simulink model "Sim_exe"  (R2020b)
settings: Solver=VariableStepAuto  StartTime=0.0  StopTime=Tf  RelTol=1e-4  AbsTol=1e-4
values from neighbouring files (symbols this model uses):
  C = [0,1]    [Main.m]
  IC_kf = zeros(2,1)    [Main.m]
  Namp = 1*10^-1    (= 0.1)    [Main.m]
  Qk = 1    [Main.m]
  Rk = 1    [Main.m]
  Tf = T(end)    [Main.m]
  Wamp = 0*5e-3    (= 0)    [Main.m]
settings Model: Creator=emanuele riva  LastModifiedBy=emanu
settings SolverCC: AutoScaleAbsTol=off
settings DataIOCC: ReturnWorkspaceOutputs=off
settings DebuggingCC: ArithmeticOperatorsInVariantConditions=warning
settings SFSimCC: SimUseLocalCustomCode=off  CustomCodeUndefinedFunction=UseInterfaceOnly
settings RTWCC: RTWUseLocalCustomCode=off
settings CodeAppCC: StateflowObjectComments=on

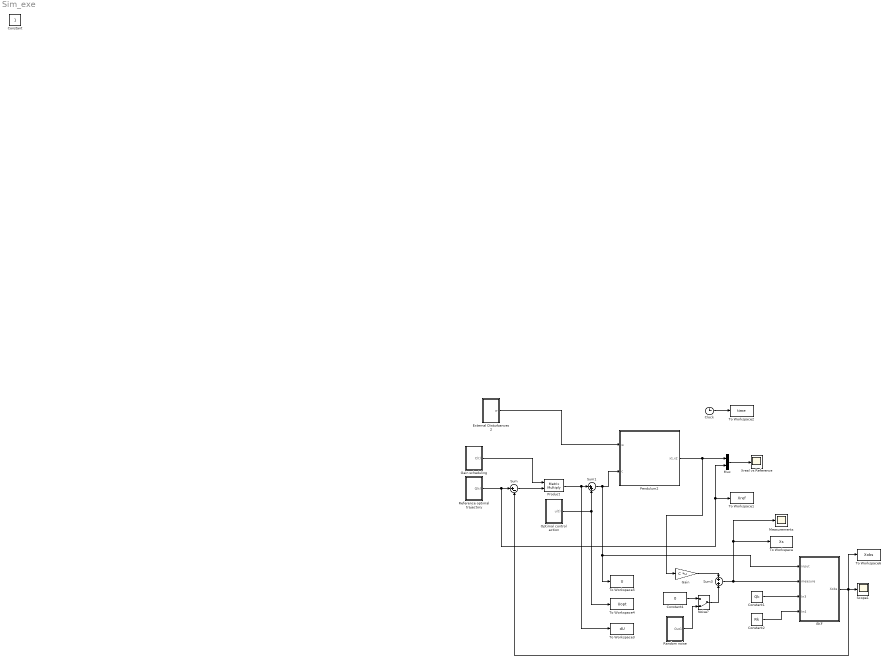
== system Sim_exe ==
  Clock : Clock
  Constant1 : Constant  Value=Qk
  Constant2 : Constant  Value=Rk
  Constant4 : Constant  Value=0
  EKF : Subsystem
  External Disturbances2 : Subsystem
  Gain : Gain  Gain=C  Multiplication=Matrix(K*u)
  Gain scheduling : Subsystem
  Measurements : Scope
  Mux : Mux  Inputs=2
  Noise? : ManualSwitch  CurrentSetting=0
  Optimal control action : Subsystem
  Pendulum2 : Subsystem
  Product : Product  Multiplication=Matrix(*)
  Random noise : Subsystem
  Reference optimal trajectory : Subsystem
  Scope1 : Scope
  Sum : Sum  Inputs=|+-
  Sum1 : Sum  Inputs=|++
  Sum3 : Sum
  To Workspace : ToWorkspace  VariableName=Xs  SaveFormat=Timeseries  SampleTime=-1
  To Workspace1 : ToWorkspace  VariableName=Xref  SaveFormat=Timeseries  SampleTime=-1
  To Workspace2 : ToWorkspace  VariableName=time  SaveFormat=Timeseries  SampleTime=-1
  To Workspace3 : ToWorkspace  VariableName=dU  SaveFormat=Timeseries  SampleTime=-1
  To Workspace4 : ToWorkspace  VariableName=Uopt  SaveFormat=Timeseries  SampleTime=-1
  To Workspace5 : ToWorkspace  VariableName=U  SaveFormat=Timeseries  SampleTime=-1
  To Workspace6 : ToWorkspace  VariableName=Xobs  SaveFormat=Timeseries  SampleTime=-1
  Xreal vs Reference : Scope
  Constant : Constant  IOType=siggen
  wires:
  Pendulum2/1(x1,x2) -> Gain/1, Mux/1
  Reference optimal trajectory/1(Q(t)) -> Mux/2, To Workspace1/1, Sum/1
  Gain scheduling/1(C(t)) -> Product/1
  Sum/1 -> Product/2
  Product/1 -> Sum1/1, To Workspace3/1
  Optimal control action/1(u(t)) -> To Workspace4/1, Sum1/2
  Mux/1 -> Xreal vs Reference/1
  Clock/1 -> To Workspace2/1
  Constant1/1 -> EKF/3(In3)
  Constant2/1 -> EKF/4(In4)
  EKF/1(Xobs) -> To Workspace6/1, Sum/2, Scope1/1
  Constant4/1 -> Noise?/1
  Random noise/1(Out1) -> Noise?/2
  Noise?/1 -> Sum3/2
  Gain/1 -> Sum3/1
  Sum3/1 -> To Workspace/1, Measurements/1, EKF/2(measure)
  Sum1/1 -> Pendulum2/2(c), To Workspace5/1, EKF/1(input)
  External Disturbances2/1(w) -> Pendulum2/1(w)

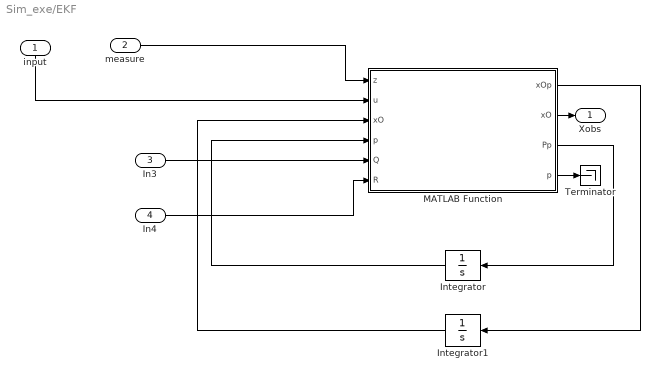
== system Sim_exe/EKF ==
  input : Inport
  measure : Inport  Port=2
  In3 : Inport  Port=3
  In4 : Inport  Port=4
  Integrator : Integrator  InitialCondition=zeros(4,1)
  Integrator1 : Integrator  InitialCondition=IC_kf
  MATLAB Function : MATLAB Function  TreatAsAtomicUnit=on
  Terminator : Terminator
  Xobs : Outport
  wires:
  MATLAB Function/1(xOp) -> Integrator1/1
  Integrator1/1 -> MATLAB Function/3("xO ")
  MATLAB Function/2(xO) -> Xobs/1
  MATLAB Function/4(p) -> Terminator/1
  input/1 -> MATLAB Function/2(u)
  In4/1 -> MATLAB Function/6(R)
  Integrator/1 -> MATLAB Function/4("p ")
  In3/1 -> MATLAB Function/5(Q)
  measure/1 -> MATLAB Function/1(z)
  MATLAB Function/3(Pp) -> Integrator/1

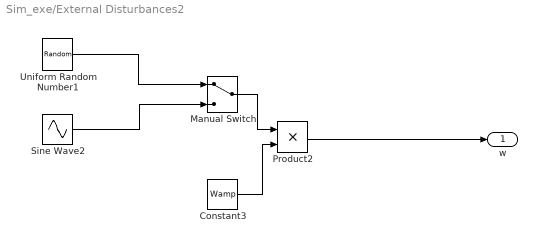
== system Sim_exe/External Disturbances2 ==
  Constant3 : Constant  Value=Wamp  VectorParams1D=off
  Manual Switch : ManualSwitch
  Product2 : Product
  Sine Wave2 : Sin  Frequency=2*pi*100  SampleTime=0  VectorParams1D=off
  Uniform Random Number1 : UniformRandomNumber  SampleTime=Tf/1000  VectorParams1D=off
  w : Outport
  wires:
  Product2/1 -> w/1
  Constant3/1 -> Product2/2
  Uniform Random Number1/1 -> Manual Switch/1
  Manual Switch/1 -> Product2/1
  Sine Wave2/1 -> Manual Switch/2

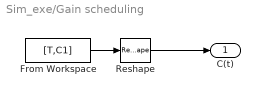
== system Sim_exe/Gain scheduling ==
  From Workspace : FromWorkspace  VariableName=[T,C1]
  Reshape : Reshape  OutputDimensionality=Row vector (2-D)
  C(t) : Outport
  wires:
  From Workspace/1 -> Reshape/1
  Reshape/1 -> C(t)/1

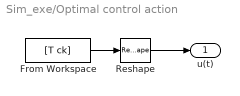
== system Sim_exe/Optimal control action ==
  From Workspace : FromWorkspace  VariableName=[T ck]
  Reshape : Reshape  OutputDimensionality=Column vector (2-D)
  u(t) : Outport
  wires:
  From Workspace/1 -> Reshape/1
  Reshape/1 -> u(t)/1

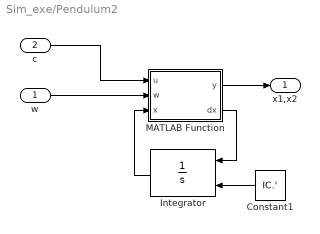
== system Sim_exe/Pendulum2 ==
  w : Inport
  c : Inport  Port=2
  Constant1 : Constant  Value=IC.'  VectorParams1D=off
  Integrator : Integrator  InitialConditionSource=external
  MATLAB Function : MATLAB Function  TreatAsAtomicUnit=on
  x1,x2 : Outport
  wires:
  w/1 -> MATLAB Function/2(w)
  c/1 -> MATLAB Function/1(u)
  MATLAB Function/1(y) -> x1,x2/1
  Constant1/1 -> Integrator/2
  Integrator/1 -> MATLAB Function/3(x)
  MATLAB Function/2(dx) -> Integrator/1

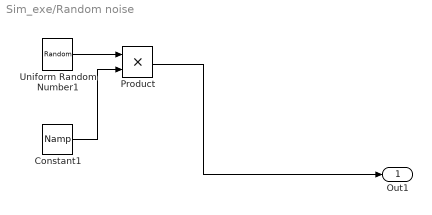
== system Sim_exe/Random noise ==
  Constant1 : Constant  Value=Namp
  Product : Product
  Uniform Random Number1 : UniformRandomNumber  Seed=19  SampleTime=0.0001  VectorParams1D=off
  Out1 : Outport
  wires:
  Product/1 -> Out1/1
  Uniform Random Number1/1 -> Product/1
  Constant1/1 -> Product/2

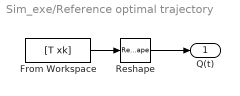
== system Sim_exe/Reference optimal trajectory ==
  From Workspace : FromWorkspace  VariableName=[T xk]
  Reshape : Reshape  OutputDimensionality=Column vector (2-D)
  Q(t) : Outport
  wires:
  From Workspace/1 -> Reshape/1
  Reshape/1 -> Q(t)/1

== matlab function Sim_exe/EKF/MATLAB Function ==
  data: z input; u input; xOp output; xO input; xO output; Pp output; p output; p input; Q input; R input
function [xOp,xO,Pp,p]  = obs(z,u,xO,p,Q,R)

Nstates = size(xO,1);

xOp = zeros(Nstates,1);
Pp = zeros(Nstates^2,1);

% Data of the pendulum
g = 9.81; % [m/s^2] gravity
L = 0.1; % [m] length of the pendulum
m = 1; % [kg] mass of the pendulum
w0 = sqrt(g/L);
zeta = 0.02;

%% Linearization around the estimated position A,C,L

% Jacobian of the dynamics
A = [ - 2*zeta*w0, - w0^2*cos(xO(2));
                1,               0];
Lm = [ 1/m/L^2; 0];

% observation matrix
C = [0,1];

%% Differential Riccati Equation - Computation of the gain matrix K

% transformation vector -> matrix
P = zeros(Nstates,Nstates);
P(1:end) = p(1:end,1);

% DRE
Out = (A*P + P*A' + Lm*Q*Lm' - P*C'*R^-1*C*P);

K = P*C'*R^-1;

% transformation matrix -> vector
Pp(1:end,1) = Out(1:end)';

%% State estimate

xOp(:,1) = [ - 2*zeta*w0*xO(1) - w0^2*sin(xO(2)) + u/m/L^2;
                                                       xO(1)];

xOp = xOp + K*(z - C*xO);

== matlab function Sim_exe/Pendulum2/MATLAB Function ==
  data: y output; dx output; u input; w input; x input
function [y,dx]  = fcn(u,w,x)

m = 1;
g = 9.81;
L = 0.1;
zeta = 0.02;
w0 = sqrt(g/L);

dx = zeros(2,1);

u = u(1) + w(1);

dx(1) = - 2*zeta*w0*x(1) - w0^2*sin(x(2)) + u/L^2/m;
dx(2) = x(1);

y = [x(1);x(2)];
